simulink library "Condensing_Boiler"  (R2016b)
settings: Solver=VariableStepAuto  StartTime=0.0  StopTime=10.0  RelTol=1e-3
libraries: carnot x4
settings Model: Creator=drhf  LastModifiedBy=drhf

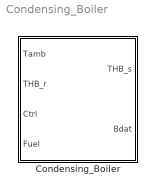
== system Condensing_Boiler ==
  Condensing_Boiler : Subsystem  mask(Condensing Boiler){Pgas=15e3, UA=0.1, vol=0.02, electricPower=[20 120], relativeQdot=[0.25 1], whichTforEfficiency=mean of inlet and outlet temperature, temperatures=[40  70], efficiency=[1.05 0.95; 1.0 0.9], lin=10, qua=100, Tini=20, nodes=1}
      mask prompts: Pgas "Heat input (= hi * GasMassflow) [W]"; UA "Heat losses in W/K"; vol "Volume (of water) in m³"; electricPower "Electric power in W (vector, index from relative power)"; relativeQdot "relative power in 0..1 (vector for row index)"; whichTforEfficiency "Efficiency table based on"; temperatures "Temperature in °C  (vector for column index)"; efficiency "Efficiency data in 0..1 (matrix)"; lin "pressure drop linear in massflow [Pa*s/kg]"; qua "pressure drop quadratic in massflow [Pa*s²/kg²]"; Tini "Initial temperature in °C"; nodes "Number of nodes"
      mask help: Multinode one-dimensional model of a boiler. Condensing effects are taken in account by an efficiency lookup table.
      mask init:
      | % set parameters UA,vol,Tini,nodes if empty
      | if isempty(UA)
      |     UA = 1;
      | end
      | if isempty(vol)
      |     vol = 0.01;
      | end
      | if isempty(Tini)
      |     Tini = 20;
      | end
      | if isempty(nodes)
      |     nodes = 20;
      | end
      mask Help: web(fullfile(path_carnot('help'),'Condensing_Boiler.html'),'-helpbrowser')
      mask TypeOptions UA: sfunBoiler/UA
      mask TypeOptions vol: sfunBoiler/vol
      mask TypeOptions whichTforEfficiency: mean of inlet and outlet temperature | inlet temperature | outlet temperature
      mask TypeOptions Tini: sfunBoiler/Tini
      mask TypeOptions nodes: sfunBoiler/nodes
      mask Display: plot(-20,0,120,100,[10,90,90,10,10],[10,10,20,20,10],[80,80,20,20],[20,90,90,20],[20,70,70,20],[24,24,30,30],[32,30,28],[30,40,30],[43,40,38],[30,40,30],[53,50,47],[30,40,30],[63,60,57],[30,40,30],[35,32,30,29,31,36,39,40,37,35],[75,69,65,58,50,49,53,59,68,75],[57,54,51,51,53,58,62,62,59,57],[76,71,67,58,49,48,54,60,69,76])

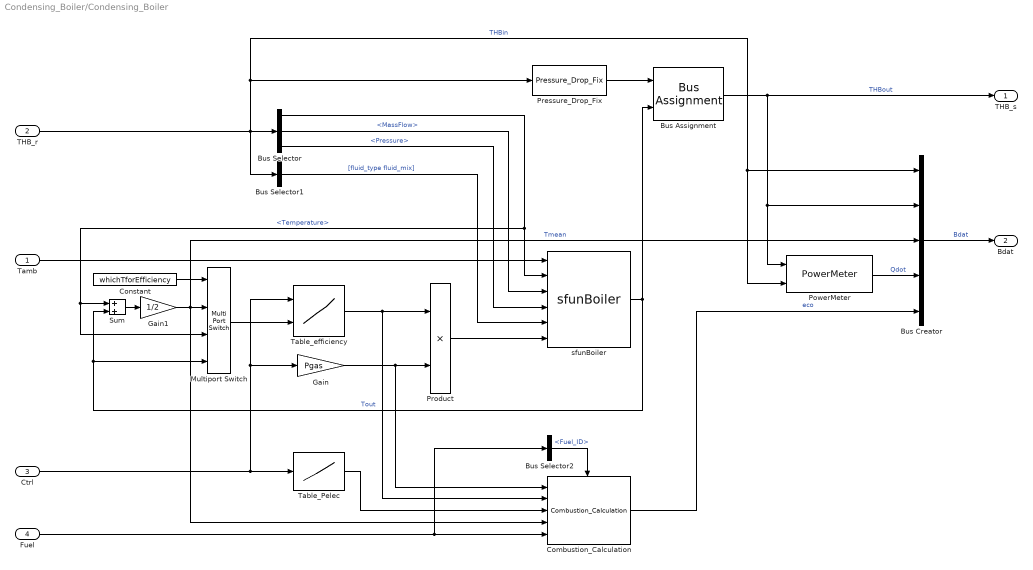
== system Condensing_Boiler/Condensing_Boiler ==
  Tamb : Inport
  THB_r : Inport  Port=2
  Ctrl : Inport  Port=3
  Fuel : Inport  Port=4
  Bus Assignment : BusAssignment  AssignedSignals=Temperature
  Bus Creator : BusCreator  Inputs=5
  Bus Selector : BusSelector  OutputSignals=Temperature,MassFlow,Pressure
  Bus Selector1 : BusSelector  OutputSignals=FluidType,FluidMix  OutputAsBus=on
  Bus Selector2 : BusSelector  OutputSignals=Fuel_ID
  Combustion_Calculation : carnot/Basic/Thermal_Models/Combustion_Calculation
  Constant : Constant  Value=whichTforEfficiency
  Gain : Gain  Gain=Pgas
  Gain1 : Gain  Gain=1/2
  Multiport Switch : MultiPortSwitch
  PowerMeter : carnot/Control/PowerMeter
  Pressure_Drop_Fix : carnot/Basic/Pressure_Drop/Pressure_Drop_Fix  con=0  lin=lin  qua=qua
  Product : Product  RndMeth=Zero
  Sum : Sum
  Table_Pelec : Lookup_n-D  NumberOfTableDimensions=1  BreakpointsForDimension1=[0 relativeQdot]  Table=[0 electricPower]  InternalRulePriority=Speed  InputSameDT=on
  Table_efficiency : Lookup_n-D  BreakpointsForDimension1=relativeQdot  BreakpointsForDimension2=temperatures  Table=efficiency  InternalRulePriority=Speed
  sfunBoiler : carnot/Basic/Thermal_Models/sfunBoiler  UA=UA  vol=vol  Tini=Tini  nodes=nodes
  THB_s : Outport
  Bdat : Outport  Port=2
  wires:
  Multiport Switch/1 -> Table_efficiency/2
  Constant/1 -> Multiport Switch/1
  Gain/1 -> Product/2, Combustion_Calculation/1
  Pressure_Drop_Fix/1 -> Bus Assignment/1
  Bus Selector2/1 -> Combustion_Calculation/Enable  "<Fuel_ID>"
  Product/1 -> sfunBoiler/6
  Ctrl/1 -> Table_Pelec/1, Gain/1, Table_efficiency/1
  Table_efficiency/1 -> Product/1, Combustion_Calculation/2
  Fuel/1 -> Bus Selector2/1, Combustion_Calculation/5
  sfunBoiler/1 -> Sum/2, Multiport Switch/4, Bus Assignment/2  "Tout"
  Bus Selector/1 -> Sum/1, Multiport Switch/3, sfunBoiler/2  "<Temperature>"
  Tamb/1 -> sfunBoiler/1
  Bus Selector/3 -> sfunBoiler/4  "<Pressure>"
  Bus Assignment/1 -> PowerMeter/1, Bus Creator/2, THB_s/1  "THBout"
  Bus Selector/2 -> sfunBoiler/3  "<MassFlow>"
  THB_r/1 -> PowerMeter/2, Bus Creator/1, Pressure_Drop_Fix/1, Bus Selector1/1, Bus Selector/1  "THBin"
  Bus Selector1/1 -> sfunBoiler/5  "[fluid_type fluid_mix]"
  Bus Creator/1 -> Bdat/1  "Bdat"
  Gain1/1 -> Combustion_Calculation/4, Multiport Switch/2, Bus Creator/3  "Tmean"
  Table_Pelec/1 -> Combustion_Calculation/3
  PowerMeter/1 -> Bus Creator/4  "Qdot"
  Combustion_Calculation/1 -> Bus Creator/5  "eco"
  Sum/1 -> Gain1/1
